simulink model "Milford"  (R2017a)
settings: Solver=FixedStepAuto  StartTime=0.0  StopTime=Cycle_End  FixedStep=0.01  MaxStep=0.01  RelTol=1e-3  EnableMultiTasking=on
PostLoadFcn:
  | , if any(exist('dsrtsu_mdlpostloadfcn', 'file') == [2, 3, 6]), try dsrtsu_mdlpostloadfcn('Execute', bdroot); catch fprintf('Error in PostLoadFcn (dsrtsu_mdlpostloadfcn) for model "%s":\n %s\n', bdroot, lasterr); end, end,
undefined symbols (not defined in the file): Actuators, APP1_OOR, APP2_OOR, APP_Mismatch, Brk_Flt, cal, ClutchEngag, DiscIntNeverNeededParam, eng, Engine, EngOverTemp, ENGTRQ_MSMCH_Degraded_CP, ENGTRQ_MSMCH_ErrCritical_CP, ENGTRQ_MSMCH_LimpHome_CP, EngTrqMismatch, ESSOverTemp, gb, Gearbox, KeyPos_Flt, lib_Actuators, lib_Sensors_2017a, lib_Transmission, Loss, LossCAN, MCUOverTemp, mot, MotDirMismatch, MotOverTemp, MotTrqMismatch, mph2kph, PRNDL_Flt, Ratio, RegenFault, Sensors, Spd, time, Transmission
libraries: simulink x110, powerlib_meascontrol x6, EC2_libraries x5, dspsigops x3, lib_Chassis x1, lib_DCDC x1, lib_Differential x1, lib_HVESS x1, lib_Engine x1, lib_OBC x1, Transmission_Validation x1, lib_Wheels x1
(part 3 of 9)

== system Milford/Sensors/CAN/EBCAN/ECM ==
  In1 : Inport
  Bus Creator : BusCreator  Inputs=7
  Bus Selector : BusSelector  OutputSignals=Sensors_to_ECM.EngActStdyStTorq_Nm,Sensors_to_ECM.EngSpd_RPM,ECM_to_Actuators.VehSpdAvgDrvn,ECM_to_Actuators.EngRunAtv,ECM_to_Actuators.Eng_Temp,ECM_to_Actuators.ECM_RollingAliveCnt
  Data Type Conversion{1..6} (6 alike) : DataTypeConversion
  ETEI_Engine_Torque_Status : Subsystem
  Ground : Ground
  PPEI_Engine_General_Status_4 : Subsystem
  PPEI_Engine_General_Status_6 : Subsystem
  PPEI_Vehicle_Speed_and_Distance : Subsystem
  PTEI_Engine_Torque_Status : Subsystem
  Out1 : Outport
  wires:
  Data Type Conversion1/1 -> Bus Creator/4  "EngRunAtv"
  Data Type Conversion3/1 -> Bus Creator/2  "EngSpd"
  PPEI_Engine_General_Status_6/1(Out1) -> Bus Creator/7
  Data Type Conversion6/1 -> PPEI_Engine_General_Status_6/1(In1)
  PPEI_Engine_General_Status_4/1(Out1) -> Bus Creator/6
  Data Type Conversion5/1 -> PPEI_Engine_General_Status_4/1(In1)
  PTEI_Engine_Torque_Status/1(Out1) -> Bus Creator/5
  Ground/1 -> PTEI_Engine_Torque_Status/1(In1)
  Bus Selector/4 -> Data Type Conversion1/1  "<EngRunAtv>"
  Bus Creator/1 -> Out1/1
  PPEI_Vehicle_Speed_and_Distance/1(Out1) -> Bus Creator/3
  ETEI_Engine_Torque_Status/1(Out1) -> Bus Creator/1
  Data Type Conversion4/1 -> PPEI_Vehicle_Speed_and_Distance/1(In1)
  Bus Selector/2 -> Data Type Conversion3/1  "<EngSpd_RPM>"
  Data Type Conversion2/1 -> ETEI_Engine_Torque_Status/1(In1)
  In1/1 -> Bus Selector/1
  Bus Selector/1 -> Data Type Conversion2/1  "<EngActStdyStTorq_Nm>"
  Bus Selector/3 -> Data Type Conversion4/1  "<VehSpdAvgDrvn>"
  Bus Selector/5 -> Data Type Conversion5/1  "<Eng_Temp>"
  Bus Selector/6 -> Data Type Conversion6/1  "<ECM_RollingAliveCnt>"

== system Milford/Sensors/CAN/HV_CAN/BMS_Hybrid ==
  In1 : Inport
  BMS_HYB_02 : Subsystem
  BMS_HYB_03 : Subsystem
  BMS_HYB_04 : Subsystem
  Bus Creator : BusCreator  Inputs=6
  Bus Selector : BusSelector  OutputSignals=BMS_HYB_02,BMS_HYB_04,BMS_HYB_03,BMS_HYB_02.BMS_Fehler_Isolation,BMS_HYB_06.BMS_Temperatur,BMS_HYB_02.BMS_Fehler_HS_verschweisst
  Data Type Conversion : DataTypeConversion
  Data Type Conversion1 : DataTypeConversion
  Data Type Conversion2 : DataTypeConversion
  Out1 : Outport
  wires:
  Data Type Conversion2/1 -> Bus Creator/6  "BMS_Fehler_HS_verschweisst"
  Bus Selector/5 -> Data Type Conversion/1  "<BMS_Temperatur>"
  Bus Selector/4 -> Data Type Conversion1/1  "<BMS_Fehler_Isolation>"
  BMS_HYB_03/1(Out1) -> Bus Creator/3
  Bus Selector/3 -> BMS_HYB_03/1(In1)  "<BMS_HYB_03>"
  BMS_HYB_04/1(Out1) -> Bus Creator/2
  BMS_HYB_02/1(Out1) -> Bus Creator/1
  Bus Creator/1 -> Out1/1
  Bus Selector/2 -> BMS_HYB_04/1(In1)  "<BMS_HYB_04>"
  Bus Selector/1 -> BMS_HYB_02/1(In1)  "<BMS_HYB_02>"
  In1/1 -> Bus Selector/1
  Data Type Conversion/1 -> Bus Creator/5  "BMS_Temperatur"
  Data Type Conversion1/1 -> Bus Creator/4  "BMS_Fehler_Isolation"
  Bus Selector/6 -> Data Type Conversion2/1  "<BMS_Fehler_HS_verschweisst>"

== system Milford/Sensors/CAN/HV_CAN/OBC ==
  In1 : Inport
  Bus Creator : BusCreator  Inputs=5
  Bus Selector : BusSelector  OutputSignals=NLG5_ACT_I,NLG5_ACT_II,NLG5_ERR,NLG5_ST,NLG5_TEMP
  NLG5_ACT_I : Subsystem
  NLG5_ACT_II : Subsystem
  NLG5_ERR : Subsystem
  NLG5_ST : Subsystem
  NLG5_TEMP : Subsystem
  Out1 : Outport
  wires:
  In1/1 -> Bus Selector/1
  Bus Selector/1 -> NLG5_ACT_I/1(In1)  "<NLG5_ACT_I>"
  NLG5_ACT_I/1(Out1) -> Bus Creator/1
  Bus Selector/2 -> NLG5_ACT_II/1(In1)  "<NLG5_ACT_II>"
  NLG5_ACT_II/1(Out1) -> Bus Creator/2
  NLG5_ERR/1(Out1) -> Bus Creator/3
  Bus Selector/3 -> NLG5_ERR/1(In1)  "<NLG5_ERR>"
  Bus Selector/4 -> NLG5_ST/1(In1)  "<NLG5_ST>"
  NLG5_ST/1(Out1) -> Bus Creator/4
  Bus Selector/5 -> NLG5_TEMP/1(In1)  "<NLG5_TEMP>"
  NLG5_TEMP/1(Out1) -> Bus Creator/5
  Bus Creator/1 -> Out1/1

== system Milford/Sensors/CAN/VEH_CAN/BCM ==
  In1 : Inport
  Bus Creator : BusCreator  Inputs=2
  Bus Selector : BusSelector  OutputSignals=SysPwrMd,BrkPdlPos
  Data Type Conversion : DataTypeConversion
  Data Type Conversion1 : DataTypeConversion
  PPEI_Brake_Apply_Status : Subsystem
  PPEI_Platfrom_General_Status : Subsystem
  Out1 : Outport
  wires:
  Data Type Conversion1/1 -> PPEI_Brake_Apply_Status/1(In1)
  Data Type Conversion/1 -> PPEI_Platfrom_General_Status/1(In1)
  Bus Creator/1 -> Out1/1
  PPEI_Brake_Apply_Status/1(Out1) -> Bus Creator/2
  PPEI_Platfrom_General_Status/1(Out1) -> Bus Creator/1
  Bus Selector/2 -> Data Type Conversion1/1  "<BrkPdlPos>"
  Bus Selector/1 -> Data Type Conversion/1  "<SysPwrMd>"
  In1/1 -> Bus Selector/1

== system Milford/Sensors/CAN/VEH_CAN/EBCM ==
  In1 : Inport
  Bus Selector : BusSelector  OutputSignals=PPEI_Chassis_General_Status_1.BrkPdlDrvAppPrsDetcd
  Constant : Constant  OutDataTypeStr=boolean
  PPEI_Chassis_General_Status_1 : Subsystem
  Terminator : Terminator
  Out1 : Outport
  wires:
  Constant/1 -> PPEI_Chassis_General_Status_1/1(In1)
  In1/1 -> Bus Selector/1
  PPEI_Chassis_General_Status_1/1(Out1) -> Out1/1
  Bus Selector/1 -> Terminator/1  "<BrkPdlDrvAppPrsDetcd>"

== system Milford/Sensors/CAN/VEH_CAN/ICCM ==
  In1 : Inport
  Out1 : Outport
  wires:
  In1/1 -> Out1/1

== system Milford/Sensors/CAN/VEH_CAN/TCM ==
  In1 : Inport
  Bus Creator : BusCreator  Inputs=4
  Bus Selector : BusSelector  OutputSignals=TCM_to _Actuator.TransEstGear,TCM_to _Actuator.LockupCmd,TCM_to _Actuator.TrnsShftLvrPos,Sensors_to_TCM.gb_trq_ratio
  Data Type Conversion{,1..3} (4 alike) : DataTypeConversion
  Out1 : Outport
  wires:
  Data Type Conversion/1 -> Bus Creator/1  "TransEstGear"
  Bus Creator/1 -> Out1/1
  In1/1 -> Bus Selector/1
  Data Type Conversion1/1 -> Bus Creator/2  "TrnsTrqCnvCltCmndMd"
  Data Type Conversion2/1 -> Bus Creator/3  "TrnsShftLvrPos"
  Data Type Conversion3/1 -> Bus Creator/4  "TrnGrRat"
  Bus Selector/1 -> Data Type Conversion/1  "<TransEstGear>"
  Bus Selector/2 -> Data Type Conversion1/1  "<LockupCmd>"
  Bus Selector/3 -> Data Type Conversion2/1  "<TrnsShftLvrPos>"
  Bus Selector/4 -> Data Type Conversion3/1  "<gb_trq_ratio>"

== system Milford/Camaro Plant Model/Transmission/Soft TCM/6L45 Logic/Gearbox_Control.Shift_Schedule.PlotShiftSchedule/Subsystem ==

== system Milford/Camaro Plant Model/Transmission/Transmission Plant/Gearbox/Inertia Calculation ==
  Inertia_in : Inport
  gear number : Inport  Port=2
  Product2 : Product  Inputs=3  SaturateOnIntegerOverflow=on  InputSameDT=on  OutDataTypeStr=Inherit: Same as first input
  Sum : Sum  Inputs=|++  SaturateOnIntegerOverflow=on  InputSameDT=on  OutDataTypeStr=Inherit: Same as first input
  Sum2 : Sum  Inputs=|++  SaturateOnIntegerOverflow=on  InputSameDT=on  OutDataTypeStr=Inherit: Same as first input
  Switch : Switch  Criteria=u2 ~= 0  Threshold=0.5  SaturateOnIntegerOverflow=on  InputSameDT=on
  gb_inertia_in : Constant  Value=Gearbox.InputShaftInertia
  gb_inertia_out : Constant  Value=Gearbox.OutputShaftInertia
  gear ratio table : Lookup  InputValues=gb.plant.init.ratio.idx1_gear  Table=gb.plant.init.ratio.map  OutDataTypeStr=double  SaturateOnIntegerOverflow=on
  Inertia : Outport
  wires:
  Switch/1 -> Inertia/1
  gear number/1 -> gear ratio table/1, Switch/2
  gb_inertia_out/1 -> Switch/3, Sum2/2
  Sum/1 -> Product2/3
  gb_inertia_in/1 -> Sum/2
  Product2/1 -> Sum2/1
  Inertia_in/1 -> Sum/1
  Sum2/1 -> Switch/1
  gear ratio table/1 -> Product2/2, Product2/1

== system Milford/Camaro Plant Model/Transmission/Transmission Plant/Gearbox/Speed Calculation ==
  gear number : Inport
  spd out : Inport  Port=2
  torque input : Inport  Port=3
  Inertia Input : Inport  Port=4
  Fcn2 : Fcn  Expr=(u[1]==0)*u[4]+(u[1]>0)*u[3]
  Mux : Mux
  P/N : Subsystem
  Product : Product  SaturateOnIntegerOverflow=on  InputSameDT=on  OutDataTypeStr=Inherit: Same as first input
  R/D : Subsystem
  gear ratio table : Lookup  InputValues=gb.plant.init.ratio.idx1_gear  Table=gb.plant.init.ratio.map  SaturateOnIntegerOverflow=on
  Speed : Outport
  wires:
  Fcn2/1 -> Speed/1
  R/D/1(spd in filtered) -> Mux/3
  P/N/1(speed) -> R/D/3(speed1), Mux/4
  Product/1 -> P/N/4(inital speed), R/D/1(spd in), Mux/2
  gear ratio table/1 -> Product/2
  spd out/1 -> Product/1
  Inertia Input/1 -> P/N/2(Inertia Input)
  torque input/1 -> P/N/1(torque input)
  gear number/1 -> gear ratio table/1, R/D/2(gear number), P/N/3(gear), Mux/1
  Mux/1 -> Fcn2/1

== system Milford/Camaro Plant Model/Transmission/Transmission Plant/Gearbox/Subsystem ==
  In1 : Inport
  In2 : Inport  Port=2
  Add : Sum
  Constant : Constant  Value=200
  Switch2 : Switch  Criteria=u2 > Threshold
  Out1 : Outport
  wires:
  Switch2/1 -> Out1/1
  In1/1 -> Add/2
  In2/1 -> Switch2/3
  [Brk_Flt] -> Switch2/2
  Constant/1 -> Add/1
  Add/1 -> Switch2/1

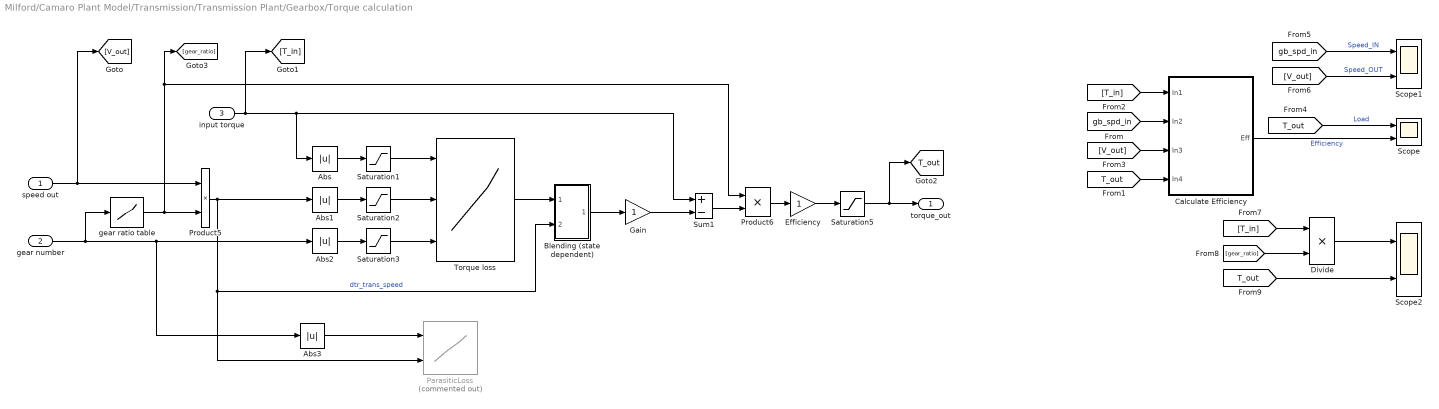
== system Milford/Camaro Plant Model/Transmission/Transmission Plant/Gearbox/Torque calculation ==
  speed out : Inport
  gear number : Inport  Port=2
  " input torque" : Inport  Port=3
  Abs : Abs  SaturateOnIntegerOverflow=on
  Abs1 : Abs  SaturateOnIntegerOverflow=on
  Abs2 : Abs  SaturateOnIntegerOverflow=on
  Abs3 : Abs
  Blending (state dependent) : Subsystem  mask(State dependent blending){xl=-gb.plant.init.spd_thr, yl=-1, xc=0, yc=0, xr=gb.plant.init.spd_thr, yr=1}
      mask prompts: xl "Left point (x):"; yl "Left point (y):"; xc "Center point (x):"; yc "Center point (y):"; xr "Right point (x):"; yr "Right point (y):"
      mask help: This block implements state dependent smoothing/blending. IMPORTANT: See help menu.
      mask Help: The output equals the product of the first input and a "hat" function defined by the three points specified in the dialog box.  The second input forms the argument to the hat function.\n\nIMPORTANT: A divide by zero error will result if first coordinates of the three points specified for the hat function are NOT distinct.
      mask Display: plot([-1 1 3 6 8], [1.5 1.5 0.5 4.0 4.0])
  Calculate Efficiency : Subsystem
  Divide : Product  Inputs=**
  Efficiency : Gain
  Gain : Gain
  ParasiticLoss : Lookup_n-D  Commented=on  BreakpointsForDimension1=Ratio  BreakpointsForDimension2=Spd  Table=Loss  InternalRulePriority=Speed  RndMeth=Simplest  InputSameDT=on
  Product5 : Product  SaturateOnIntegerOverflow=on  InputSameDT=on  OutDataTypeStr=Inherit: Same as first input
  Product6 : Product  SaturateOnIntegerOverflow=on  InputSameDT=on  OutDataTypeStr=Inherit: Same as first input
  Saturation1 : Saturate  UpperLimit=inf  LowerLimit=min( gb.plant.init.trq_loss.idx1_trq )
  Saturation2 : Saturate  UpperLimit=inf  LowerLimit=min( gb.plant.init.trq_loss.idx2_spd )
  Saturation3 : Saturate  UpperLimit=8  LowerLimit=1
  Saturation5 : Saturate  UpperLimit=inf  LowerLimit=min( gb.plant.init.trq_loss.idx1_trq )
  Scope : Scope  NumInputPorts=2
  Scope1 : Scope  NumInputPorts=2
  Scope2 : Scope  NumInputPorts=2
  Sum1 : Sum  Inputs=+-  SaturateOnIntegerOverflow=on  InputSameDT=on  OutDataTypeStr=Inherit: Same as first input
  Torque loss : Lookup_n-D  NumberOfTableDimensions=3  BreakpointsForDimension1=gb.plant.init.trq_loss.idx1_trq  BreakpointsForDimension2=gb.plant.init.trq_loss.idx2_spd  BreakpointsForDimension3=gb.plant.init.trq_loss.idx3_gear  Table=gb.plant.init.trq_loss.map
  gear ratio table : Lookup  InputValues=gb.plant.init.ratio.idx1_gear  Table=gb.plant.init.ratio.map  SaturateOnIntegerOverflow=on
  torque_out : Outport
  tag scope: T_out=global
  wires:
  Saturation5/1 -> [T_out], torque_out/1
  [T_out] -> Scope2/2
  Divide/1 -> Scope2/1
  [gear_ratio] -> Divide/2
  [T_in] -> Divide/1
  [V_out] -> Scope1/2  "Speed_OUT"
  [gb_spd_in] -> Scope1/1  "Speed_IN"
  [T_out] -> Scope/1  "Load"
  [V_out] -> Calculate Efficiency/3(In3)
  Calculate Efficiency/1(Eff) -> Scope/2  "Efficiency"
  [T_out] -> Calculate Efficiency/4(In4)
  [gb_spd_in] -> Calculate Efficiency/2(In2)
  [T_in] -> Calculate Efficiency/1(In1)
  Torque loss/1 -> Blending (state dependent)/1(Input)
  Gain/1 -> Sum1/2
  Efficiency/1 -> Saturation5/1
  Abs3/1 -> ParasiticLoss/1
  Saturation3/1 -> Torque loss/3
  Abs2/1 -> Saturation3/1
  gear ratio table/1 -> Product6/1, [gear_ratio], Product5/2
  gear number/1 -> gear ratio table/1, Abs2/1, Abs3/1
  " input torque"/1 -> Abs/1, Sum1/1, [T_in]
  Sum1/1 -> Product6/2
  Blending (state dependent)/1(Output) -> Gain/1
  Product6/1 -> Efficiency/1
  speed out/1 -> Product5/1, [V_out]
  Abs1/1 -> Saturation2/1
  Product5/1 -> Abs1/1, Blending (state dependent)/2(Control (state)), ParasiticLoss/2  "dtr_trans_speed"
  Abs/1 -> Saturation1/1
  Saturation1/1 -> Torque loss/1
  Saturation2/1 -> Torque loss/2

== system Milford/Controller_with_Transmission_Manager1/HSC/Camaro Fault Detection/Component Diagnostic/Driver Input Diagnostic ==
  note: APP1
      | APP2
      | BPP
      | Driver Component Status
      |
      | 1
      | 1
      | 1
      | 1
      |
      | 0
      | 1
      | 1
      | 1
      |
      | 1
      | 0
      | 1
      | 1
      |
      | 0
      | 0
      | 1
      | 0
      |
      | 1
      | 1
      | 0
      | 0
      |
      | 0
      | 0
      | 0
      | 0
  note: Driver_CompStatus
      | 1 = Component Online
      | 0 = Component Offline
  In1 : Inport
  Bus Selector : BusSelector  OutputSignals=Driver_SigDiag.Drv_APP1_[%]_SigValid,Driver_SigDiag.Drv_APP2_[%]_SigValid,Driver_SigDiag.Drv_APP_Agree,Driver_SigDiag.Drv_BPP_[%]_SigValid,Driver_SigDiag.Drv_KeyPos_[0 3]_SigValid,Driver_SigDiag.Drv_PRNDL_SigValid,Driver_SigDiag.Brake_Failed
  Driver_Input_Diag : Stateflow chart  TreatAsAtomicUnit=on
  Logical Operator : Logic  Inputs=3  AllPortsSameDT=off  OutDataTypeStr=boolean
  Out1 : Outport
  wires:
  Bus Selector/7 -> Driver_Input_Diag/5(BrakeFail)  "<Brake_Failed>"
  Bus Selector/6 -> Driver_Input_Diag/4(PRNDL)  "<Drv_PRNDL_SigValid>"
  Bus Selector/5 -> Driver_Input_Diag/3(KeyPos)  "<Drv_KeyPos_[0 3]_SigValid>"
  Bus Selector/3 -> Logical Operator/3  "<Drv_APP_Agree>"
  Logical Operator/1 -> Driver_Input_Diag/1(APP_Valid)  "APP_Valid"
  Driver_Input_Diag/1(Driver_Input_Status) -> Out1/1  "Driver_Input_Status"
  Bus Selector/4 -> Driver_Input_Diag/2(Drv_BPP_SigValid)  "<Drv_BPP_[%]_SigValid>"
  Bus Selector/2 -> Logical Operator/2  "<Drv_APP2_[%]_SigValid>"
  Bus Selector/1 -> Logical Operator/1  "<Drv_APP1_[%]_SigValid>"
  In1/1 -> Bus Selector/1

== system Milford/Controller_with_Transmission_Manager1/HSC/Camaro Fault Detection/Component Diagnostic/ESS Component Diagnostic ==
  note: (Need modify)
  In1 : Inport
  BMS_CompDiag1 : Stateflow chart  TreatAsAtomicUnit=on
  Bus Selector : BusSelector  OutputSignals=ESS_SigDiag.BMS_RollingAliveActive_SigValid,ESS_SigDiag.BMS_contactorsFailed_Detected,ESS_SigDiag.BMS_essTemp_[degC]_SigValid,ESS_SigDiag.essTempRange[0_4],ESS_SigDiag.BMS_essSOC_0_1_SigValid,ESS_SigDiag.essTempRange[0_4],ESS_SigDiag.essCur_A_SigValid,ESS_SigDiag.BMSgdf_SigValid,Driver_SigDiag.Drv_KeyPos_[0 3]_SigValid
  Compare To Zero : simulink/Logic and Bit Operations/Compare To Zero  relop===  OutDataTypeStr=boolean
  Data Type Conversion : DataTypeConversion
  HVessFltReset : Constant
  Logical Operator : Logic  Operator=OR  AllPortsSameDT=off  OutDataTypeStr=boolean
  Logical Operator1 : Logic  AllPortsSameDT=off  OutDataTypeStr=boolean
  Terminator : Terminator
  Terminator1 : Terminator
  Out1 : Outport
  wires:
  [contactorsFailed_Detected] -> Logical Operator1/1
  Logical Operator1/1 -> BMS_CompDiag1/6(ess_GroundFault)
  Bus Selector/8 -> Logical Operator1/2  "<BMSgdf_SigValid>"
  Logical Operator/1 -> BMS_CompDiag1/7(ClearFault)
  HVessFltReset/1 -> Logical Operator/2
  Compare To Zero/1 -> Logical Operator/1
  Bus Selector/9 -> Compare To Zero/1  "<Drv_KeyPos_[0 3]_SigValid>"
  Bus Selector/7 -> BMS_CompDiag1/5(essCur_A_SigValid)  "<essCur_A_SigValid>"
  Bus Selector/6 -> Terminator1/1  "<essTempRange[0_4]>"
  Bus Selector/5 -> BMS_CompDiag1/4(BMS_essSOC_0_1_SigValid)  "<BMS_essSOC_0_1_SigValid>"
  Data Type Conversion/1 -> BMS_CompDiag1/3(BMS_essTemp_SigValid)  "BMS_essTemp_SigValid"
  Bus Selector/3 -> Data Type Conversion/1  "<BMS_essTemp_[degC]_SigValid>"
  Bus Selector/4 -> Terminator/1  "<essTempRange[0_4]>"
  BMS_CompDiag1/1(BMS_Status) -> Out1/1  "BMS_Status"
  Bus Selector/2 -> BMS_CompDiag1/2(BMS_contactorsFailed_SigValid), [contactorsFailed_Detected]  "<BMS_contactorsFailed_Detected>"
  Bus Selector/1 -> BMS_CompDiag1/1(BMS_RollingAliveActive_SigValid)  "<BMS_RollingAliveActive_SigValid>"
  In1/1 -> Bus Selector/1

== system Milford/Controller_with_Transmission_Manager1/HSC/Camaro Fault Detection/Component Diagnostic/Engine Component Diagnostic ==
  note: Notes
  note: 0: component needs to be offline
      | 1: component needs torque plant to deliver creep torque
      | 2: component needs torque plant to limit maximum torque delivery
      | 3: component needs torque plant to operate normally
  note: add the temperature, mismatch torquesignal and have different status to the component
  note: Eng_tempRange
      | 1: normal
      | 2: high range
      | 3:above max
  note: ENGTRQ_MSMCH_Degraded_CP (40Nm): ENGTRQ_Degraded fault code.
      | ENGTRQ_MSMCH_LimpHome_CP (70Nm): ENGTRQ_LimpHome
      | ENGTRQ_MSMCH_ErrCritical_CP (100Nm): ENGTRQ_ErrCritical
  note: Eng_Torq_MsmchLevel
      | 1:Normal torque
      | 2: Limit max power
      | 3: Deliver creep torque
      | 4: offline
  In1 : Inport
  Bus Selector : BusSelector  OutputSignals=Engine_SigDiag.ECMRollingAliveActive,Engine_SigDiag.engTrqCmdRecvd_SigValid,Engine_SigDiag.ECMTrqCmd_Nm,Engine_SigDiag.EngActStdyStTorq_Nm,Engine_SigDiag.EngRunAtValid,Engine_SigDiag.Engine_Speed_rpm_SigValid,Engine_SigDiag.Eng_TempValid,Engine_SigDiag.Eng_TempRange[123],Driver_SigDiag.Drv_KeyPos_[0 3]_SigValid
  Bus Selector1 : BusSelector  OutputSignals=Eng_Torque_Mismch_Critical
  Compare To Zero : simulink/Logic and Bit Operations/Compare To Zero  relop===  OutDataTypeStr=boolean
  ECM_CompDiag : Stateflow chart  TreatAsAtomicUnit=on
  Eng_FltReset : Constant
  Eng_Torq_MsmchLevel : Stateflow chart  Commented=on  TreatAsAtomicUnit=on
  Logical Operator : Logic  Operator=OR  AllPortsSameDT=off  OutDataTypeStr=boolean
  Override  engTrqCmd : Subsystem
  Terminator1 : Terminator
  TorqMismatch Detection : Subsystem
  Out1 : Outport
  Out2 : Outport  Port=2
  wires:
  Override  engTrqCmd/1(Out1) -> ECM_CompDiag/2(engTrqCmdRecvd_SigValid)
  Bus Selector1/1 -> ECM_CompDiag/3(Eng_Torq_Msmch)  "<Eng_Torque_Mismch_Critical>"
  TorqMismatch Detection/1(Eng_Torque_Mismch) -> Out2/1, Bus Selector1/1  "EngTrqMismchType"
  Bus Selector/5 -> TorqMismatch Detection/3(In3)  "<EngRunAtValid>"
  Bus Selector/4 -> TorqMismatch Detection/2(In2)  "<EngActStdyStTorq_Nm>"
  Bus Selector/3 -> TorqMismatch Detection/1(In1)  "<ECMTrqCmd_Nm>"
  Bus Selector/8 -> ECM_CompDiag/5(Eng_TempRange_123)  "<Eng_TempRange[123]>"
  Bus Selector/7 -> Terminator1/1  "<Eng_TempValid>"
  Bus Selector/9 -> Compare To Zero/1  "<Drv_KeyPos_[0 3]_SigValid>"
  Logical Operator/1 -> ECM_CompDiag/6(ClearFault)
  Eng_FltReset/1 -> Logical Operator/2
  Compare To Zero/1 -> Logical Operator/1
  ECM_CompDiag/1(ECM_Status) -> Out1/1  "ECM_Status"
  Bus Selector/6 -> ECM_CompDiag/4(Engine_Speed_rpm_SigValid)  "<Engine_Speed_rpm_SigValid>"
  Bus Selector/2 -> Override  engTrqCmd/1(In1)  "<engTrqCmdRecvd_SigValid>"
  Bus Selector/1 -> ECM_CompDiag/1(ECM_RollingAliveActive)  "<ECMRollingAliveActive>"
  In1/1 -> Bus Selector/1

== system Milford/Controller_with_Transmission_Manager1/HSC/Camaro Fault Detection/Component Diagnostic/Override Driver Status ==
  note: Override Switch Subsystem
  note: This subsystem is used to override the model value of a signal to a constant value
  In1 : Inport
  Data Type Conversion3 : DataTypeConversion
  Override Value : Constant  OutDataTypeStr=double
  Override_Driver_Status : Constant  Value=0
  Switch : Switch  Criteria=u2 > Threshold
  Out1 : Outport
  wires:
  Data Type Conversion3/1 -> Switch/3
  Override Value/1 -> Switch/1
  Switch/1 -> Out1/1
  In1/1 -> Data Type Conversion3/1
  Override_Driver_Status/1 -> Switch/2

== system Milford/Controller_with_Transmission_Manager1/HSC/Camaro Fault Detection/Component Diagnostic/Override ESS Status ==
  note: Override Switch Subsystem
  note: This subsystem is used to override the model value of a signal to a constant value
  In1 : Inport
  Data Type Conversion3 : DataTypeConversion
  Override Value : Constant  Value=2  OutDataTypeStr=double
  Override_ESS_Status : Constant  Value=0
  Switch : Switch  Criteria=u2 > Threshold
  Terminator : Terminator
  Out1 : Outport
  wires:
  Data Type Conversion3/1 -> Switch/3
  Override Value/1 -> Switch/1, Out1/1
  Override_ESS_Status/1 -> Switch/2
  In1/1 -> Data Type Conversion3/1
  Switch/1 -> Terminator/1

== system Milford/Controller_with_Transmission_Manager1/HSC/Camaro Fault Detection/Component Diagnostic/Override Engine Status ==
  note: Override Switch Subsystem
  note: This subsystem is used to override the model value of a signal to a constant value
  In1 : Inport
  Data Type Conversion3 : DataTypeConversion
  Override Value1 : Constant  Value=2  OutDataTypeStr=double
  Override_Engine_Status : Constant  Value=0
  Switch : Switch  Criteria=u2 > Threshold
  Terminator : Terminator
  Out1 : Outport
  wires:
  Data Type Conversion3/1 -> Switch/3
  Override_Engine_Status/1 -> Switch/2
  Override Value1/1 -> Switch/1, Out1/1
  In1/1 -> Data Type Conversion3/1
  Switch/1 -> Terminator/1

== system Milford/Controller_with_Transmission_Manager1/HSC/Camaro Fault Detection/Component Diagnostic/Override TCM Status ==
  note: Override Switch Subsystem
  note: This subsystem is used to override the model value of a signal to a constant value
  In1 : Inport
  Data Type Conversion3 : DataTypeConversion
  Override Value1 : Constant  Value=2  OutDataTypeStr=double
  Override_TCM_Status : Constant  Value=0
  Switch : Switch  Criteria=u2 > Threshold
  Out1 : Outport
  wires:
  Data Type Conversion3/1 -> Switch/3
  Override Value1/1 -> Switch/1
  Override_TCM_Status/1 -> Switch/2
  Switch/1 -> Out1/1
  In1/1 -> Data Type Conversion3/1

== system Milford/Controller_with_Transmission_Manager1/HSC/Camaro Fault Detection/Component Diagnostic/Transmission Component Diagnostic ==
  In1 : Inport
  Bus Selector : BusSelector  OutputSignals=Transmission_SigDiag.TCMRollingAliveActive_SigValid,Transmission_SigDiag.LvrPosTrnsShft_SigValid,Transmission_SigDiag.TransEstGear_SigValid,Transmission_SigDiag.LockupCmd_SigValid,Transmission_SigDiag.VehDirFault
  TCM_CompDia : Stateflow chart  TreatAsAtomicUnit=on
  Out1 : Outport
  wires:
  Bus Selector/5 -> TCM_CompDia/5(VehDirFault)  "<VehDirFault>"
  TCM_CompDia/1(TCM_Status) -> Out1/1  "TCM_Status"
  Bus Selector/4 -> TCM_CompDia/4(LockupCmd_SigValid)  "<LockupCmd_SigValid>"
  Bus Selector/3 -> TCM_CompDia/3(TransEstGear_SigValid)  "<TransEstGear_SigValid>"
  Bus Selector/2 -> TCM_CompDia/2(LvrPosTrnsShft_SigValid)  "<LvrPosTrnsShft_SigValid>"
  Bus Selector/1 -> TCM_CompDia/1(TCMRollingAliveActive_SigValid)  "<TCMRollingAliveActive_SigValid>"
  In1/1 -> Bus Selector/1

== system Milford/Controller_with_Transmission_Manager1/HSC/Camaro Fault Detection/Input Conversions/BMS_Conversions ==
  note: BMS: Conversions and Override Switches
      | (Battery Management System)
  note: hvBattVolt_V
  note: hvBusVolt_V
  note: 5: error
  note: 1 : Error Insulation
  note: MO_BMS_Sollmodus
      | The battery mode is requested:
      | 0: Standby; communication active
      | 1: HV power enable / normal driving mode
      | 2: Balancing Mode
      | 3: HV power enable / external_load_external start
      | 4: HV power enable / external load_EV_PlugIn
      | 5: None
  note: BMS_IstModus
      | actual state of the battery / Current status of the battery
      | 0 : Standby ; communication active
      | 1 : main contactors closed / HV power activated / normal driving
      | 2 : closed / Balancing mode main contactors activated
      | 3 : external charging via charger High
      | 4 : external charging HV
      | 5 : Error Battery
      | 6 : External DC Charging HV
      | 7 : Init
  note: Fehler_HS_verschweisst
      | 1 : Error: Main contactor welded
  In1 : Inport
  Bus Creator : BusCreator  Inputs=11
  Bus Selector : BusSelector  OutputSignals=from_CAN.fromHV_CAN.from_BMSHybrid.BMS_HYB_02.BMS_HYB_02_BZ,from_CAN.fromHV_CAN.from_BMSHybrid.BMS_HYB_02.BMS_IstModus,from_CAN.fromHV_CAN.from_BMSHybrid.BMS_HYB_02.BMS_IstStrom,from_CAN.fromHV_CAN.from_BMSHybrid.BMS_SOC,from_CAN.fromHV_CAN.from_BMSHybrid.BMS_HYB_02.BMS_IstSpannung,from_CAN.fromHV_CAN.from_BMSHybrid.BMS_Spannung_ZwKr,from_CAN.fromHV_CAN.from_BMSHybrid.BMS_Temperatur,from_CAN.fromHV_CAN.from_BMSHybrid.BMS_Fehler_Isolation,from_CAN.fromHV_CAN.from_BMSHybrid.BMS_HYB_02.BMS_Fehler_HS_offen,from_CAN.fromHV_CAN.from_BMSHybrid.BMS_Fehler_HS_verschweisst
  Conversion  BMS_gdf : DataTypeConversion  OutDataTypeStr=boolean
  Conversion  Fehler_HS_offen : DataTypeConversion  OutDataTypeStr=boolean
  Conversion  Fehler_HS_verschweisst : DataTypeConversion  OutDataTypeStr=boolean
  Conversion  closeContactorsCmd : DataTypeConversion  OutDataTypeStr=boolean
  Conversion  contactorsClsd : DataTypeConversion  OutDataTypeStr=boolean
  Conversion  essTemp_K : DataTypeConversion  OutDataTypeStr=double
  Conversion  hvBattVolt_V : DataTypeConversion  OutDataTypeStr=double
  Conversion  hvBusVolt_V : DataTypeConversion  OutDataTypeStr=double
  Conversion  rollingAliveCnt : DataTypeConversion  OutDataTypeStr=int8
  Conversion essCur_A : DataTypeConversion  OutDataTypeStr=double
  Conversion essSOC_0_1 : DataTypeConversion  OutDataTypeStr=double
  K to C : Bias  Bias=-273.15
  Override  BMS_gdf 0_1 : Subsystem
  Override  closeContactorsCmd : Subsystem
  Override  contactorsClsd : Subsystem
  Override  essCur_A : Subsystem
  Override  essSOC_0_1 : Subsystem
  Override  essTemp_C : Subsystem
  Override  hvBattVolt_V : Subsystem
  Override  hvBusVolt_V : Subsystem
  Override  rollingAliveCnt [1_3] : Subsystem
  Override Fehler_HS_offen : Subsystem
  Override Fehler_HS_verschweisst : Subsystem
  Out1 : Outport
  wires:
  Override Fehler_HS_verschweisst/1(Out1) -> Bus Creator/11  "Fehler_HS_verschweisst"
  Conversion  Fehler_HS_verschweisst/1 -> Override Fehler_HS_verschweisst/1(In1)
  Bus Selector/10 -> Conversion  Fehler_HS_verschweisst/1  "<BMS_Fehler_HS_verschweisst>"
  Override Fehler_HS_offen/1(Out1) -> Bus Creator/10  "Fehler_HS_offen"
  Conversion  Fehler_HS_offen/1 -> Override Fehler_HS_offen/1(In1)
  Bus Selector/9 -> Conversion  Fehler_HS_offen/1  "<BMS_Fehler_HS_offen>"
  [MO_BMS_Sollmodus] -> Conversion  closeContactorsCmd/1
  Bus Selector/6 -> Conversion  hvBusVolt_V/1  "<BMS_Spannung_ZwKr>"
  Bus Selector/1 -> Conversion  rollingAliveCnt/1  "<BMS_HYB_02_BZ>"
  Bus Selector/3 -> Conversion essCur_A/1  "<BMS_IstStrom>"
  Bus Selector/4 -> Conversion essSOC_0_1/1  "<BMS_SOC>"
  Bus Selector/5 -> Conversion  hvBattVolt_V/1  "<BMS_IstSpannung>"
  Bus Selector/8 -> Conversion  BMS_gdf/1  "<BMS_Fehler_Isolation>"
  Bus Selector/7 -> Conversion  essTemp_K/1  "<BMS_Temperatur>"
  Bus Selector/2 -> Conversion  contactorsClsd/1  "<BMS_IstModus>"
  Override  BMS_gdf 0_1/1(Out1) -> Bus Creator/9  "BMS_gdf"
  Conversion  BMS_gdf/1 -> Override  BMS_gdf 0_1/1(In1)
  K to C/1 -> Override  essTemp_C/1(In1)
  Override  essTemp_C/1(Out1) -> Bus Creator/8  "essTemp_C"
  Conversion  essTemp_K/1 -> K to C/1
  Override  hvBusVolt_V/1(Out1) -> Bus Creator/7  "hvBusVolt_V"
  Override  essCur_A/1(Out1) -> Bus Creator/4  "essCur_A"
  Override  hvBattVolt_V/1(Out1) -> Bus Creator/6  "hvBattVolt_V"
  Override  essSOC_0_1/1(Out1) -> Bus Creator/5  "essSOC_0_1"
  Override  contactorsClsd/1(Out1) -> Bus Creator/3  "contactorsClsd"
  Conversion  hvBusVolt_V/1 -> Override  hvBusVolt_V/1(In1)
  Conversion  hvBattVolt_V/1 -> Override  hvBattVolt_V/1(In1)
  Conversion essSOC_0_1/1 -> Override  essSOC_0_1/1(In1)
  Conversion essCur_A/1 -> Override  essCur_A/1(In1)
  Conversion  contactorsClsd/1 -> Override  contactorsClsd/1(In1)
  Override  closeContactorsCmd/1(Out1) -> Bus Creator/2  "MO_BMS_Sollmodus [0-5]"
  Conversion  closeContactorsCmd/1 -> Override  closeContactorsCmd/1(In1)
  Bus Creator/1 -> Out1/1  "BMS_Conv"
  Override  rollingAliveCnt [1_3]/1(Out1) -> Bus Creator/1  "BMSrollingAliveCnt [123]"
  Conversion  rollingAliveCnt/1 -> Override  rollingAliveCnt [1_3]/1(In1)
  In1/1 -> Bus Selector/1

== system Milford/Controller_with_Transmission_Manager1/HSC/Camaro Fault Detection/Input Conversions/DriverInput_Conversions ==
  note: Driver Controls: Conversions and Override Switches
  note: SysPwrMd (EC3)
      | 0 - Off
      | 1 -  Accessory
      | 2 - Run
      | 3 - Crank Request
  In1 : Inport
  Bus Creator : BusCreator  Inputs=7
  Bus Selector : BusSelector  OutputSignals=from_Analog.Driver_APP1,from_Analog.Driver_APP2,from_CAN.fromVEH_CAN.from_BCM.BrkPdlPos,from_CAN.fromVEH_CAN.from_BCM.SysPwrMd,from_CAN.fromVEH_CAN.from_TCM.TrnsShftLvrPos,from_CAN.fromEBCAN.from_ECM.VehSpdAvgDrvn,from_Digital.SW_Regen_Disable
  Conversion  APP1 (%) : DataTypeConversion  OutDataTypeStr=double
  Conversion  APP2 (%) : DataTypeConversion  OutDataTypeStr=double
  Conversion  BPP (%) : DataTypeConversion  OutDataTypeStr=double
  Conversion  KeyPos [0_3] : DataTypeConversion  OutDataTypeStr=int8
  Conversion  V [mph] : DataTypeConversion  OutDataTypeStr=double
  Conversion PRNDL : DataTypeConversion  OutDataTypeStr=uint8
  Conversion Regen : DataTypeConversion  OutDataTypeStr=uint8
  Override  KeyPos [0_3] : Subsystem
  Override APP (%) : Subsystem
  Override APP (%)1 : Subsystem
  Override BPP (%) : Subsystem
  Override PRNDL : Subsystem
  Override Regen : Subsystem
  Override V [mph] : Subsystem
  Out1 : Outport
  wires:
  Override Regen/1(Out1) -> Bus Creator/7  "SW_Regen"
  Conversion Regen/1 -> Override Regen/1(In1)
  Bus Selector/7 -> Conversion Regen/1  "<SW_Regen_Disable>"
  Override V [mph]/1(Out1) -> Bus Creator/6  "V [mph]"
  Conversion  V [mph]/1 -> Override V [mph]/1(In1)
  Bus Selector/6 -> Conversion  V [mph]/1  "<VehSpdAvgDrvn>"
  Conversion  APP2 (%)/1 -> Override APP (%)1/1(In1)
  Override APP (%)1/1(Out1) -> Bus Creator/2  "APP2[%]"
  Bus Selector/5 -> Conversion PRNDL/1  "<TrnsShftLvrPos>"
  Bus Selector/2 -> Conversion  APP2 (%)/1  "<Driver_APP2>"
  Override PRNDL/1(Out1) -> Bus Creator/5  "PRNDL"
  Conversion PRNDL/1 -> Override PRNDL/1(In1)
  Conversion  BPP (%)/1 -> Override BPP (%)/1(In1)
  Bus Creator/1 -> Out1/1  "DriverControls_Conv"
  Override  KeyPos [0_3]/1(Out1) -> Bus Creator/4  "keyPos [0_3]"
  Override BPP (%)/1(Out1) -> Bus Creator/3  "BPP [%]"
  Conversion  KeyPos [0_3]/1 -> Override  KeyPos [0_3]/1(In1)
  Bus Selector/4 -> Conversion  KeyPos [0_3]/1  "<SysPwrMd>"
  Bus Selector/3 -> Conversion  BPP (%)/1  "<BrkPdlPos>"
  Bus Selector/1 -> Conversion  APP1 (%)/1  "<Driver_APP1>"
  Override APP (%)/1(Out1) -> Bus Creator/1  "APP1 [%]"
  Conversion  APP1 (%)/1 -> Override APP (%)/1(In1)
  In1/1 -> Bus Selector/1

== system Milford/Controller_with_Transmission_Manager1/HSC/Camaro Fault Detection/Input Conversions/ECM_Conversions ==
  note: ECM: Input Conversions and Override Switches
      | (Engine and ECM)
  In1 : Inport
  Bus Creator : BusCreator  Inputs=6
  Bus Selector : BusSelector  OutputSignals=from_CAN.fromEBCAN.from_ECM.PlatEngSpdCmdStARC,from_CAN.fromEBCAN.from_ECM.EngSpd,from_CAN.fromEBCAN.from_ECM.EngCltTmp,from_CAN.fromEBCAN.from_ECM.EngRunAtv,from_CAN.fromEBCAN.from_ECM.EngActStdyStTorq
  Conversion  ECMTrqCmd_Nm : DataTypeConversion  OutDataTypeStr=double
  Conversion  EngActStdyStTorq_Nm : DataTypeConversion  OutDataTypeStr=double
  Conversion  EngRunAtv : DataTypeConversion  OutDataTypeStr=boolean
  Conversion  Engine_Speed_rpm : DataTypeConversion  OutDataTypeStr=double
  Conversion  Engine_Temp[DegC] : DataTypeConversion  OutDataTypeStr=double
  Conversion  rollingAliveCnt : DataTypeConversion  OutDataTypeStr=int8
  Memory : Memory
  Override  ECMTrqCmd_Nm : Subsystem
  Override  ECMrollingAliveCnt : Subsystem
  Override  EngActStdyStTorq_Nm : Subsystem
  Override  EngRunAtv : Subsystem
  Override  EngineSpeed_rpm : Subsystem
  Override  Engine_Temp[DegC] : Subsystem
  Out1 : Outport
  wires:
  Memory/1 -> Conversion  ECMTrqCmd_Nm/1
  [AxlEngTrqCmd] -> Memory/1
  Bus Selector/1 -> Conversion  rollingAliveCnt/1  "<PlatEngSpdCmdStARC>"
  Override  EngActStdyStTorq_Nm/1(Out1) -> Bus Creator/6  "EngActStdyStTorq_Nm"
  Override  EngRunAtv/1(Out1) -> Bus Creator/5  "EngRunAtv"
  Override  Engine_Temp[DegC]/1(Out1) -> Bus Creator/4  "Engine_Temp[DegC]"
  Conversion  EngActStdyStTorq_Nm/1 -> Override  EngActStdyStTorq_Nm/1(In1)
  Conversion  EngRunAtv/1 -> Override  EngRunAtv/1(In1)
  Conversion  Engine_Temp[DegC]/1 -> Override  Engine_Temp[DegC]/1(In1)
  Bus Selector/5 -> Conversion  EngActStdyStTorq_Nm/1  "<EngActStdyStTorq>"
  Bus Selector/4 -> Conversion  EngRunAtv/1  "<EngRunAtv>"
  Bus Selector/3 -> Conversion  Engine_Temp[DegC]/1  "<EngCltTmp>"
  Override  EngineSpeed_rpm/1(Out1) -> Bus Creator/3  "EngineSpeed_rpm"
  Conversion  Engine_Speed_rpm/1 -> Override  EngineSpeed_rpm/1(In1)
  Bus Selector/2 -> Conversion  Engine_Speed_rpm/1  "<EngSpd>"
  Conversion  ECMTrqCmd_Nm/1 -> Override  ECMTrqCmd_Nm/1(In1)
  Override  ECMTrqCmd_Nm/1(Out1) -> Bus Creator/2  "ECMTrqCmd_Nm"
  Bus Creator/1 -> Out1/1  "ECM_Conv"
  Override  ECMrollingAliveCnt/1(Out1) -> Bus Creator/1  "ECMrollingAliveCnt [123]"
  Conversion  rollingAliveCnt/1 -> Override  ECMrollingAliveCnt/1(In1)
  In1/1 -> Bus Selector/1

== system Milford/Controller_with_Transmission_Manager1/HSC/Camaro Fault Detection/Input Conversions/TCM_Conversions ==
  note: TCM: Input Conversions and Override Switches
      | (Transmission Control Module)
  In1 : Inport
  Bus Creator : BusCreator  Inputs=4
  Bus Selector : BusSelector  OutputSignals=from_CAN.fromVEH_CAN.from_TCM.TrnsShftLvrPos,from_CAN.fromVEH_CAN.from_TCM.TransEstGear,from_CAN.fromVEH_CAN.from_TCM.TrnsTrqCnvCltCmndMd
  Conversion  LockupCmd : DataTypeConversion  OutDataTypeStr=boolean
  Conversion  LvrPosTrnsShft : DataTypeConversion  OutDataTypeStr=int8
  Conversion  TransEstGear : DataTypeConversion  OutDataTypeStr=int8
  Conversion  rollingAliveCnt : DataTypeConversion  OutDataTypeStr=int8
  Override  LockupCmd : Subsystem
  "Override  LvrPosTrnsShft " : Subsystem
  Override  TransEstGear : Subsystem
  Override  rollingAliveCnt [123] : Subsystem
  TCM_RollinAliveCounter : Subsystem
  Out1 : Outport
  wires:
  TCM_RollinAliveCounter/1(Out1) -> Conversion  rollingAliveCnt/1
  In1/1 -> Bus Selector/1
  Conversion  rollingAliveCnt/1 -> Override  rollingAliveCnt [123]/1(In1)
  Override  rollingAliveCnt [123]/1(Out1) -> Bus Creator/1  "TCMrollingAliveCnt [123]"
  Bus Creator/1 -> Out1/1  "TCM_Conv"
  Bus Selector/1 -> Conversion  LvrPosTrnsShft/1  "<TrnsShftLvrPos>"
  "Override  LvrPosTrnsShft "/1(Out1) -> Bus Creator/2  "LvrPosTrnsShft"
  Conversion  LvrPosTrnsShft/1 -> "Override  LvrPosTrnsShft "/1(In1)
  Bus Selector/2 -> Conversion  TransEstGear/1  "<TransEstGear>"
  Conversion  TransEstGear/1 -> Override  TransEstGear/1(In1)
  Override  TransEstGear/1(Out1) -> Bus Creator/3  "TransEstGear"
  Bus Selector/3 -> Conversion  LockupCmd/1  "<TrnsTrqCnvCltCmndMd>"
  Conversion  LockupCmd/1 -> Override  LockupCmd/1(In1)
  Override  LockupCmd/1(Out1) -> Bus Creator/4  "LockupCmd_0_1"

== system Milford/Controller_with_Transmission_Manager1/HSC/Camaro Fault Detection/Signal Diagnostic/Driver Signal Diagnostic ==
  note: Driver Controls : Signal Diagnostic
  Sensors1 : Inport
  APP_Crosscheck : Subsystem
  AccPedalValidity : Stateflow chart  TreatAsAtomicUnit=on
  AccPedalValidity1 : Stateflow chart  TreatAsAtomicUnit=on
  BPP_faild_ovrd : Constant  Value=0  OutDataTypeStr=boolean
  BrakeFailureDetection : Subsystem
  Bus Creator : BusCreator  Inputs=7
  Bus Selector : BusSelector  OutputSignals=DriverControls_Conv.APP1 [%],DriverControls_Conv.APP2[%],DriverControls_Conv.BPP [%],DriverControls_Conv.V [mph],DriverControls_Conv.keyPos [0_3],DriverControls_Conv.PRNDL
  ClearAPP1fault : Constant  Value=0
  ClearAPP2fault : Constant  Value=0
  Constant2 : Constant  Value=0
  Constant3 : Constant  OutDataTypeStr=boolean
  Conversion  APP1 (%)1 : DataTypeConversion  OutDataTypeStr=boolean
  Conversion  APP1 (%)2 : DataTypeConversion
  Conversion  APP1 (%)3 : DataTypeConversion
  Drv_APP1_valid_ovrd : Constant  Value=0  OutDataTypeStr=boolean
  Drv_APP2_valid_ovrd : Constant  Value=0  OutDataTypeStr=boolean
  Interval Test : simulink/Logic and Bit Operations/Interval Test  IntervalClosedRight=on  uplimit=100  IntervalClosedLeft=on  lowlimit=0  OutDataTypeStr=boolean
  Interval Test1 : simulink/Logic and Bit Operations/Interval Test  IntervalClosedRight=on  uplimit=3  IntervalClosedLeft=on  lowlimit=0  OutDataTypeStr=boolean
  Interval Test2 : simulink/Logic and Bit Operations/Interval Test  IntervalClosedRight=on  uplimit=4  IntervalClosedLeft=on  lowlimit=0  OutDataTypeStr=boolean
  Latch : Subsystem
  Latch1 : Subsystem
  Logical Operator1 : Logic  AllPortsSameDT=off  OutDataTypeStr=boolean
  Logical Operator5 : Logic  Operator=OR  AllPortsSameDT=off  OutDataTypeStr=boolean
  Logical Operator6 : Logic  Operator=OR  AllPortsSameDT=off  OutDataTypeStr=boolean
  Pulse Generator : DiscretePulseGenerator  PulseType=Time based  Period=0.1  PulseWidth=10
  Scope : Scope
  Driver_SigDiag : Outport
  wires:
  Pulse Generator/1 -> Scope/1, BrakeFailureDetection/Trigger
  BPP_faild_ovrd/1 -> Logical Operator1/1
  Latch1/1(Out1) -> Logical Operator1/2  "Brake_Failed"
  Logical Operator1/1 -> Conversion  APP1 (%)2/1  "Brake_Failed"
  Latch/1(Drv_APP_Agree) -> Conversion  APP1 (%)3/1  "Drv_APP_Agree"
  Interval Test1/1 -> Bus Creator/6  "Drv_KeyPos_[0 3]_SigValid"
  Conversion  APP1 (%)2/1 -> Bus Creator/5  "Brake_Failed"
  Conversion  APP1 (%)3/1 -> Bus Creator/3  "Drv_APP_Agree"
  AccPedalValidity/1(signalValid) -> Logical Operator6/2  "Drv_APP1_[%]_SigValid"
  Drv_APP1_valid_ovrd/1 -> Logical Operator6/1
  AccPedalValidity1/1(signalValid) -> Logical Operator5/2  "Drv_APP2_[%]_SigValid"
  Drv_APP2_valid_ovrd/1 -> Logical Operator5/1
  Interval Test2/1 -> Bus Creator/7  "Drv_PRNDL_SigValid"
  BrakeFailureDetection/1(DecelFail) -> Latch1/1(In1)  "Brake_Failed"
  Conversion  APP1 (%)1/1 -> Latch1/2(In2)
  Constant2/1 -> Conversion  APP1 (%)1/1
  Bus Selector/4 -> BrakeFailureDetection/2(VehSpeed)  "<V [mph]>"
  APP_Crosscheck/1(Out1) -> Latch/1(In1)  "Drv_APP_Agree"
  Constant3/1 -> Latch/2(In2)
  Bus Selector/6 -> Interval Test2/1  "<PRNDL>"
  Bus Creator/1 -> Driver_SigDiag/1  "Driver_SignalDiag"
  Logical Operator5/1 -> Bus Creator/2  "Drv_APP2_[%]_SigValid"
  Interval Test/1 -> Bus Creator/4  "Drv_BPP_[%]_SigValid"
  Logical Operator6/1 -> Bus Creator/1  "Drv_APP1_[%]_SigValid"
  Bus Selector/5 -> Interval Test1/1  "<keyPos [0_3]>"
  Bus Selector/3 -> BrakeFailureDetection/1(BPP), Interval Test/1  "<BPP [%]>"
  ClearAPP2fault/1 -> AccPedalValidity1/1(clearFaults)
  ClearAPP1fault/1 -> AccPedalValidity/1(clearFaults)
  Bus Selector/2 -> APP_Crosscheck/2(In2), AccPedalValidity1/2(signalValue)  "<APP2[%]>"
  Bus Selector/1 -> APP_Crosscheck/1(In1), AccPedalValidity/2(signalValue)  "<APP1 [%]>"
  Sensors1/1 -> Bus Selector/1

== system Milford/Controller_with_Transmission_Manager1/HSC/Camaro Fault Detection/Signal Diagnostic/ESS Signal Diagnostic ==
  note: BMS : Signal Diagnostic
  note: 1) Rolling alive detection : is the component on and transmitting?
      | 2) Probably move the voltage check to component diagnostic (no signal from Bosch to check the contactors status)
      | 3) Is  the T signal within an acceptable range?
  note: SOC Range check definition :
      | 0 = below normal operation (<0.15)
      | 1 = low range ([0.15 0.30])
      | 2 = normal range (0.3)
      | 3= SOC high/full (>0.95)
  note: Temperature Range check :
      | 0 = below normal operation (<-28)
      | 1 = low range (<0 - >-28)
      | 2 = normal range (0 -30 C)
      | 3= high range (>30)
      | 4= above max value allowed (>55)
  note: Error: contactors welded,Contactors don't close when commanded
  note: max charge current: 180A
      | Max discharge current: 315A;
  Sensors1 : Inport
  Bus Creator : BusCreator  Inputs=14
  Bus Selector : BusSelector  OutputSignals=BMS_Conv.BMSrollingAliveCnt [123],BMS_Conv.hvBattVolt_V,BMS_Conv.hvBusVolt_V,BMS_Conv.Fehler_HS_offen,BMS_Conv.MO_BMS_Sollmodus [0-5],BMS_Conv.Fehler_HS_verschweisst,BMS_Conv.essTemp_C,BMS_Conv.essSOC_0_1,BMS_Conv.essCur_A,BMS_Conv.BMS_gdf
  Contactors status check : Subsystem
  ESS SOC Validity Check : Subsystem
  ESS Temp Validity Check : Subsystem
  Interval Test : simulink/Logic and Bit Operations/Interval Test  IntervalClosedRight=on  uplimit=180  IntervalClosedLeft=on  lowlimit=-315  OutDataTypeStr=boolean
  Interval Test1 : simulink/Logic and Bit Operations/Interval Test  IntervalClosedRight=on  uplimit=7  IntervalClosedLeft=on  lowlimit=0  OutDataTypeStr=boolean
  Interval Test2 : simulink/Logic and Bit Operations/Interval Test  IntervalClosedRight=on  uplimit=430  IntervalClosedLeft=on  lowlimit=291  OutDataTypeStr=boolean
  Logical Operator : Logic  Operator=OR  AllPortsSameDT=off  OutDataTypeStr=boolean
  Max charging voltage fault detect : Subsystem
  Override_ BMS_RACvalid1 : Constant  Value=0
  Rolling Alive Counter Detection : Subsystem
  Validity Check : Subsystem
  ESS_SigDiag : Outport
  wires:
  Override_ BMS_RACvalid1/1 -> Logical Operator/1
  Rolling Alive Counter Detection/1(Out1) -> Logical Operator/2  "BMS_RollingAliveActive_SigValid"
  [BusVolt] -> Bus Creator/3  "hvBusVolt_V"
  Max charging voltage fault detect/1(Out1) -> Bus Creator/5  "ChargVoltFlt"
  [BusVolt] -> Max charging voltage fault detect/1(In1)
  [BattVolt] -> Contactors status check/1(In1)
  Interval Test2/1 -> Bus Creator/2  "OverVolt_Detected"
  Interval Test1/1 -> Bus Creator/6  "Contatctors_Status_Validity"
  Bus Selector/5 -> Interval Test1/1  "<MO_BMS_Sollmodus [0-5]>"
  Bus Selector/6 -> Bus Creator/7  "<Fehler_HS_verschweisst>"
  Contactors status check/1(Out1) -> Bus Creator/4  "BMS_contactorsFailed_Detected"
  Bus Selector/4 -> Contactors status check/3(In3)  "<Fehler_HS_offen>"
  Bus Selector/3 -> [BusVolt], Contactors status check/2(In2)  "<hvBusVolt_V>"
  ESS Temp Validity Check/2(Out2) -> Bus Creator/9
  ESS Temp Validity Check/1(Out1) -> Bus Creator/8
  Bus Selector/7 -> ESS Temp Validity Check/1(In1)  "<essTemp_C>"
  ESS SOC Validity Check/2(Out2) -> Bus Creator/11
  ESS SOC Validity Check/1(Out1) -> Bus Creator/10
  Bus Selector/8 -> ESS SOC Validity Check/1(In1)  "<essSOC_0_1>"
  Validity Check/1(Out1) -> Bus Creator/13  "BMSgdf_SigValid"
  Bus Selector/10 -> Validity Check/1(In1), Bus Creator/14  "<BMS_gdf>"
  Interval Test/1 -> Bus Creator/12  "essCur_A_SigValid"
  Bus Selector/9 -> Interval Test/1  "<essCur_A>"
  Bus Creator/1 -> ESS_SigDiag/1  "ESS_SignalDiag"
  Bus Selector/2 -> [BattVolt], Interval Test2/1  "<hvBattVolt_V>"
  Logical Operator/1 -> Bus Creator/1  "BMS_RollingAliveActive_SigValid"
  Bus Selector/1 -> Rolling Alive Counter Detection/1(In1)  "<BMSrollingAliveCnt [123]>"
  Sensors1/1 -> Bus Selector/1

== system Milford/Controller_with_Transmission_Manager1/HSC/Camaro Fault Detection/Signal Diagnostic/Engine Signal Diagnostic ==
  note: Engine_Temp:
      | Normal range: <100
      | above max:>120
      | Limited range: 100-120
  note: ECM : Signal Diagnostic
  Sensors1 : Inport
  Bus Creator : BusCreator  Inputs=9
  Bus Selector : BusSelector  OutputSignals=ECM_Conv.ECMrollingAliveCnt [123],ECM_Conv.ECMTrqCmd_Nm,ECM_Conv.EngActStdyStTorq_Nm,ECM_Conv.EngineSpeed_rpm,ECM_Conv.Engine_Temp[DegC],ECM_Conv.EngRunAtv
  Constant1 : Constant
  EngTempValidity_Check : Subsystem
  Engine_Temp[DegC] : Stateflow chart  TreatAsAtomicUnit=on
  Interval Test : simulink/Logic and Bit Operations/Interval Test  IntervalClosedRight=on  uplimit=233  IntervalClosedLeft=on  lowlimit=0  OutDataTypeStr=boolean
  Interval Test1 : simulink/Logic and Bit Operations/Interval Test  IntervalClosedRight=on  uplimit=6500  IntervalClosedLeft=on  lowlimit=0  OutDataTypeStr=boolean
  Interval Test2 : simulink/Logic and Bit Operations/Interval Test  IntervalClosedRight=on  uplimit=233  IntervalClosedLeft=on  lowlimit=0  OutDataTypeStr=boolean
  Interval Test3 : simulink/Logic and Bit Operations/Interval Test  IntervalClosedRight=on  uplimit=1  IntervalClosedLeft=on  lowlimit=0  OutDataTypeStr=boolean
  Rolling Alive Counter Detection1 : Subsystem
  Engine_SigDiag : Outport
  wires:
  EngTempValidity_Check/1(Out1) -> Bus Creator/7  "Eng_TempValid"
  Engine_Temp[DegC]/1(EngTempRange) -> Bus Creator/8, EngTempValidity_Check/1(In1)  "Eng_TempRange[123]"
  Constant1/1 -> Engine_Temp[DegC]/1(clearFaults)
  Interval Test3/1 -> Bus Creator/9  "EngRunAtValid"
  Bus Selector/6 -> Interval Test3/1  "<EngRunAtv>"
  Bus Selector/5 -> Engine_Temp[DegC]/2(Engine_Temp_DegC)  "<Engine_Temp[DegC]>"
  Interval Test2/1 -> Bus Creator/4  "EngActStdyStTorq_SigValid"
  Bus Selector/3 -> Interval Test2/1, Bus Creator/5  "<EngActStdyStTorq_Nm>"
  Interval Test1/1 -> Bus Creator/6  "Engine_Speed_rpm_SigValid"
  Bus Selector/4 -> Interval Test1/1  "<EngineSpeed_rpm>"
  Bus Creator/1 -> Engine_SigDiag/1  "Engine_SignalDiag"
  Interval Test/1 -> Bus Creator/3  "engTrqCmdRecvd_SigValid"
  Bus Selector/2 -> Interval Test/1, Bus Creator/2  "<ECMTrqCmd_Nm>"
  Rolling Alive Counter Detection1/1(Out1) -> Bus Creator/1  "ECMRollingAliveActive"
  Bus Selector/1 -> Rolling Alive Counter Detection1/1(In1)  "<ECMrollingAliveCnt [123]>"
  Sensors1/1 -> Bus Selector/1

== system Milford/Controller_with_Transmission_Manager1/HSC/Camaro Fault Detection/Signal Diagnostic/Subsystem1 ==
  note: Signal Naming Rule
      | Example: xxx_yyy_[z]_SigValid
      | xxx: source of the signal (Drv, Clu, BCM, ECM, TCM, BMS and MCU)
      | yyy: description of the signal
      | z: unit of the signal (V, A, Nm, m/s, %, 01, 0123, etc.)
  note: Signal Valid Setting Rule
      | xxx_yyy_[z]_SigValid could be 0 or 1
      | 0: signal invalid
      | 1: signal vaild

== system Milford/Controller_with_Transmission_Manager1/HSC/Camaro Fault Detection/Signal Diagnostic/Transmission Signal Diagnostic ==
  note: Lever Position:
      | 1 P
      | 2 R
      | 3 N
      | 4 D
      | 0: L
  note: TransEstGear
      | 0 : Not Supported
      | 1 : First Gear
      | 2 : Second Gear
      | 3 : Third Gear
      | 4 : Fourth Gear
      | 5 : Fifth Gear
      | 6 : Sixth Gear
      | 7 : Seventh Gear
      | 8 : Eight Gear
      | 10: EVT Mode 1
      | 11: EVT Mode 2
      | 12: CVT Forward Gear
      | 13: Neutral Gear
      | 14: Reverse Gear
      | 15: Park Gear
  note: TCM : Signal Diagnostic
  Sensors1 : Inport
  Bus Creator : BusCreator  Inputs=5
  Bus Selector : BusSelector  OutputSignals=TCM_Conv.TCMrollingAliveCnt [123],TCM_Conv.LvrPosTrnsShft,TCM_Conv.TransEstGear,DriverControls_Conv.V [mph],TCM_Conv.LockupCmd_0_1
  Interval Test : simulink/Logic and Bit Operations/Interval Test  IntervalClosedRight=on  uplimit=4  IntervalClosedLeft=on  lowlimit=0  OutDataTypeStr=boolean
  Interval Test1 : simulink/Logic and Bit Operations/Interval Test  IntervalClosedRight=on  uplimit=15  IntervalClosedLeft=on  lowlimit=0  OutDataTypeStr=boolean
  Interval Test2 : simulink/Logic and Bit Operations/Interval Test  IntervalClosedRight=on  uplimit=1  IntervalClosedLeft=on  lowlimit=0  OutDataTypeStr=boolean
  Rolling Alive Counter Detection : Subsystem
  Vehicle Direction Fault Detection : Subsystem
  Out2 : Outport
  wires:
  Vehicle Direction Fault Detection/1(Out1) -> Bus Creator/4  "VehDirFault"
  Interval Test2/1 -> Bus Creator/5  "LockupCmd_SigValid"
  Interval Test1/1 -> Bus Creator/3  "TransEstGear_SigValid"
  Interval Test/1 -> Bus Creator/2  "LvrPosTrnsShft_SigValid"
  Bus Selector/5 -> Interval Test2/1  "<LockupCmd_0_1>"
  Bus Selector/3 -> Interval Test1/1  "<TransEstGear>"
  Bus Selector/2 -> Interval Test/1, Vehicle Direction Fault Detection/1(LvrPosTrnsShft)  "<LvrPosTrnsShft>"
  Bus Creator/1 -> Out2/1
  Rolling Alive Counter Detection/1(Out1) -> Bus Creator/1  "TCMRollingAliveActive_SigValid"
  Bus Selector/1 -> Rolling Alive Counter Detection/1(In1)  "<TCMrollingAliveCnt [123]>"
  Sensors1/1 -> Bus Selector/1
  Bus Selector/4 -> Vehicle Direction Fault Detection/2(Speed)  "<V [mph]>"
